simulink model "WindFarm_2023_BaseModel_v2"  (R2019a)
(part 3 of 27)

  5 km fault6/RConn1 -- Wind Type IV Detailed v2.1 - 7/LConn1
  5 km fault6/RConn2 -- Wind Type IV Detailed v2.1 - 7/LConn2
  5 km fault6/RConn3 -- Wind Type IV Detailed v2.1 - 7/LConn3
  5 km fault14/LConn1 -- 5 km fault5/RConn1
  5 km fault14/LConn2 -- 5 km fault5/RConn2
  5 km fault14/LConn3 -- 5 km fault5/RConn3
  5 km fault15/RConn2 -- 5 km fault9/LConn2
  5 km fault16/LConn1 -- 5 km fault9/RConn1
  5 km fault15/RConn1 -- 5 km fault9/LConn1
  5 km fault15/RConn3 -- 5 km fault9/LConn3
  5 km fault16/LConn2 -- 5 km fault9/RConn2
  5 km fault16/LConn3 -- 5 km fault9/RConn3
  Three-Phase Series RLC Load9/LConn3 -- Three-Phase Breaker 3/LConn3 -- Bus380kVOnshoreSubstation/RConn3
  Three-Phase Series RLC Load9/LConn2 -- Three-Phase Breaker 3/LConn2 -- Bus380kVOnshoreSubstation/RConn2
  Three-Phase Breaker 3/RConn1 -- 5 km fault3/LConn1 -- Three-Phase Breaker 6/LConn1
  Bus380kVOnshore2/RConn2 -- Three-Phase Series RLC Load3/LConn2 -- 5 km fault10/LConn2
  5 km fault10/LConn3 -- Three-Phase Series RLC Load3/LConn3 -- Bus380kVOnshore2/RConn3
  Bus380kVOnshore2/RConn1 -- Three-Phase Series RLC Load3/LConn1 -- 5 km fault10/LConn1
  5 km fault10/RConn1 -- Three-Phase Series RLC Load2/LConn1 -- Bus380kVSubA38_2/LConn1
  5 km fault10/RConn2 -- Three-Phase Series RLC Load2/LConn2 -- Bus380kVSubA38_2/LConn2
  5 km fault10/RConn3 -- Three-Phase Series RLC Load2/LConn3 -- Bus380kVSubA38_2/LConn3
  5 km fault7/RConn1 -- Wind Type IV Detailed v2.1 - 6/LConn1
  5 km fault7/RConn2 -- Wind Type IV Detailed v2.1 - 6/LConn2
  5 km fault7/RConn3 -- Wind Type IV Detailed v2.1 - 6/LConn3
  Bus380kVSubA38_4/RConn1 -- 5 km fault7/LConn1
  Bus380kVSubA38_4/RConn2 -- 5 km fault7/LConn2
  Bus380kVSubA38_4/RConn3 -- 5 km fault7/LConn3
  5 km fault13/RConn1 -- Bus_Fault1/LConn3 -- 5 km fault11/LConn1
  5 km fault13/RConn2 -- Bus_Fault1/LConn2 -- 5 km fault11/LConn2
  5 km fault13/RConn3 -- Bus_Fault1/LConn1 -- 5 km fault11/LConn3
  1Bus380kVSubB8/RConn1 -- 5 km fault4/LConn1
  1Bus380kVSubB8/RConn2 -- 5 km fault4/LConn2
  1Bus380kVSubB8/RConn3 -- 5 km fault4/LConn3
  5 km fault14/RConn1 -- Bus380kVOnshore3/LConn1
  5 km fault14/RConn2 -- Bus380kVOnshore3/LConn2
  5 km fault14/RConn3 -- Bus380kVOnshore3/LConn3
  5 km fault16/RConn1 -- Bus380kVOnshore4/LConn1
  5 km fault16/RConn2 -- Bus380kVOnshore4/LConn2
  5 km fault16/RConn3 -- Bus380kVOnshore4/LConn3
  Three-Phase Transformer Inductance Matrix Type (Three Windings)1/LConn2 -- Bus380kVOnshore4/RConn2
  Bus380kVOnshore4/RConn1 -- Three-Phase Transformer Inductance Matrix Type (Three Windings)1/LConn1
  Bus380kVOnshore4/RConn3 -- Three-Phase Transformer Inductance Matrix Type (Three Windings)1/LConn3
  Three-Phase Transformer Inductance Matrix Type (Three Windings)4/LConn2 -- Bus380kVOnshore3/RConn2
  Bus380kVOnshore3/RConn1 -- Three-Phase Transformer Inductance Matrix Type (Three Windings)4/LConn1
  Bus380kVOnshore3/RConn3 -- Three-Phase Transformer Inductance Matrix Type (Three Windings)4/LConn3
  Three-Phase Transformer Inductance Matrix Type (Three Windings)4/RConn1 -- Bus380kVOnshore1/LConn1
  Three-Phase Transformer Inductance Matrix Type (Three Windings)4/RConn2 -- Bus380kVOnshore1/LConn2
  Three-Phase Transformer Inductance Matrix Type (Three Windings)4/RConn3 -- Bus380kVOnshore1/LConn3
  Three-Phase Transformer Inductance Matrix Type (Three Windings)1/RConn1 -- Bus380kVOnshore2/LConn1
  Three-Phase Transformer Inductance Matrix Type (Three Windings)1/RConn2 -- Bus380kVOnshore2/LConn2
  Three-Phase Transformer Inductance Matrix Type (Three Windings)1/RConn3 -- Bus380kVOnshore2/LConn3
  Three-Phase Breaker 2/LConn1 -- 5 km fault11/RConn1
  Three-Phase Breaker 2/LConn2 -- 5 km fault11/RConn2
  Three-Phase Breaker 2/LConn3 -- 5 km fault11/RConn3
  5 km fault13/LConn1 -- Three-Phase Breaker 1/RConn1
  Three-Phase Breaker 1/RConn2 -- 5 km fault13/LConn2
  Three-Phase Breaker 1/RConn3 -- 5 km fault13/LConn3
  Ground3/LConn1 -- "Grounding Transformer "/RConn1
  Ground4/LConn1 -- Grounding Transformer 1/RConn1
  Ground5/LConn1 -- Grounding Transformer 2/RConn1
  1Bus380kVSubB3/RConn1 -- Three-Phase Fault1/LConn1
  1Bus380kVSubB3/RConn2 -- Three-Phase Fault1/LConn2
  1Bus380kVSubB3/RConn3 -- Three-Phase Fault1/LConn3
  Bus_Fault1/RConn3 -- 1Bus380kVSubB3/LConn3
  Bus_Fault1/RConn2 -- 1Bus380kVSubB3/LConn2
  Bus_Fault1/RConn1 -- 1Bus380kVSubB3/LConn1
  Three-Phase Series RLC Load9/LConn1 -- Three-Phase Breaker 3/LConn1 -- Bus380kVOnshoreSubstation/RConn1
  Three-Phase Breaker 3/RConn2 -- 5 km fault3/LConn2 -- Three-Phase Breaker 6/LConn2
  Three-Phase Breaker 3/RConn3 -- 5 km fault3/LConn3 -- Three-Phase Breaker 6/LConn3
  Three-Phase Breaker 6/RConn2 -- 5 km fault15/LConn2
  5 km fault15/LConn1 -- Three-Phase Breaker 6/RConn1
  5 km fault15/LConn3 -- Three-Phase Breaker 6/RConn3
  Three-Phase Breaker 7/LConn2 -- 5 km fault3/RConn2
  Three-Phase Breaker 7/RConn2 -- 5 km fault5/LConn2
  Three-Phase Breaker 7/RConn1 -- 5 km fault5/LConn1
  Three-Phase Breaker 7/LConn1 -- 5 km fault3/RConn1
  5 km fault3/RConn3 -- Three-Phase Breaker 7/LConn3
  Three-Phase Breaker 7/RConn3 -- 5 km fault5/LConn3
  Three-Phase Breaker 8/LConn2 -- 5 km fault12/RConn2
  5 km fault12/RConn1 -- Three-Phase Breaker 8/LConn1
  5 km fault12/RConn3 -- Three-Phase Breaker 8/LConn3
